simulink subsystem "HP_FirstOrder"  (R2024b)
settings: Solver=VariableStepAuto  StartTime=0.0  StopTime=10.0  RelTol=1e-3
settings Model: Creator=mykola  LastModifiedBy=nick

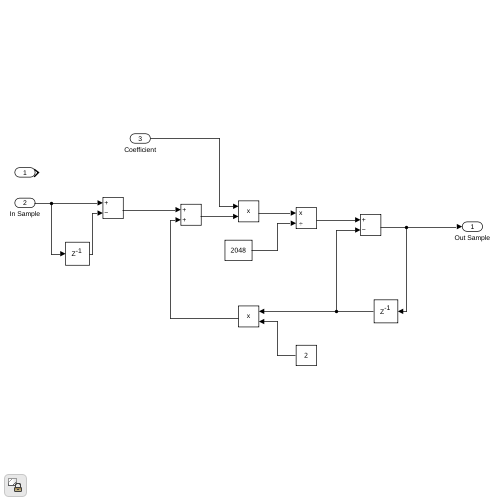
[thumbnail: Simulink's stored preview of the top-level diagram]
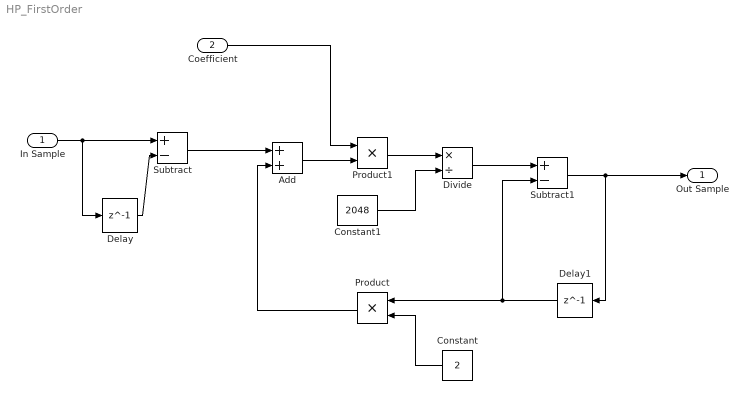
== system HP_FirstOrder ==
  In Sample : Inport
  Coefficient : Inport  Port=2
  Add : Sum
  Constant : Constant  Value=2
  Constant1 : Constant  Value=2048
  Delay : Delay  DelayLength=1
  Delay1 : Delay  DelayLength=1
  Divide : Product  Inputs=*/
  Product : Product
  Product1 : Product
  Subtract : Sum  Inputs=+-
  Subtract1 : Sum  Inputs=+-  OutDataTypeStr=int16
  Out Sample : Outport
  wires:
  In Sample/1 -> Subtract/1, Delay/1
  Delay/1 -> Subtract/2
  Subtract/1 -> Add/1
  Constant/1 -> Product/2
  Product/1 -> Add/2
  Subtract1/1 -> Delay1/1, Out Sample/1
  Delay1/1 -> Product/1, Subtract1/2
  Add/1 -> Product1/2
  Divide/1 -> Subtract1/1
  Product1/1 -> Divide/1
  Constant1/1 -> Divide/2
  Coefficient/1 -> Product1/1
